simulink model "file_changed_port"  (R2021a)
settings: Solver=FixedStepDiscrete  StartTime=0.0  StopTime=10.0  RelTol=1e-3
CloseFcn:
  | try
  | rmdir slprj\ s
  | catch
  | end
  | try
  | folder_name = [bdroot '*'];
  | rmdir(folder_name,'s')
  | catch
  | end
  | try
  | file_temp_name = [bdroot '.slxc'];
  | delete(file_temp_name)
  | catch
  | end
  | clear folder_name file_temp_name
settings Model: Creator=Administrator  LastModifiedBy=Administrator
settings DataIOCC: SaveOutput=off  SignalLogging=off  DSMLogging=off  SaveTime=off  ReturnWorkspaceOutputs=off
settings OptimizationCC: DefaultParameterBehavior=Inlined  EnhancedBackFolding=on  PassReuseOutputArgsAs=Individual arguments  ZeroExternalMemoryAtStartup=off  ZeroInternalMemoryAtStartup=off  OptimizeBlockOrder=speed  DifferentSizesBufferReuse=on  OptimizationCustomize=off  EfficientTunableParamExpr=on
settings DebuggingCC: ParameterTunabilityLossMsg=error
settings SFSimCC: MATLABDynamicMemAlloc=off
settings RTWCC: SystemTargetFile=ert.tlc  GenCodeOnly=on  TemplateMakefile=ert_default_tmf  GenerateReport=on  LaunchReport=on
settings CodeAppCC: ForceParamTrailComments=on  IgnoreCustomStorageClasses=off  OperatorAnnotations=on  SimulinkDataObjDesc=on  SFDataObjDesc=on  InsertBlockDesc=on
settings ERTTargetCC: TargetLangStandard=C99 (ISO)  GenerateSampleERTMain=on  InlinedParameterPlacement=NonHierarchical  ERTCustomFileTemplate=example_file_process.tlc

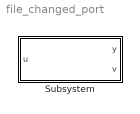
== system file_changed_port ==
  Subsystem : Subsystem  mask{gain=0, P=on}
      mask prompts: P "Sel"
      mask Callback P:
      | userdata = get(gcbh,'userdata');
      | state = get(gcbh,'P');
      | if ~strcmp(state,userdata)
      |         if strcmp(state,'on')
      |             replace_block([get(gcbh,'Parent') '/' get(gcbh, 'Name')],'Name', 'y','Outport','noprompt')
      |             set_param([gcb '/y'],'Port','1')
      |         end
      |         if strcmp(state,'off')
      |             replace_block([get(gcbh,'Parent') '/' get(gcbh, 'Name')],'Name', 'y','Terminator','noprompt')
      |         end
      | end
      | set(gcbh,'userdata',state);

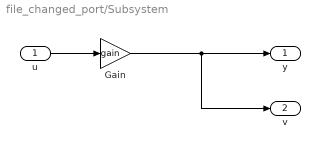
== system file_changed_port/Subsystem ==
  u : Inport
  Gain : Gain  Gain=gain
  y : Outport
  v : Outport  Port=2
  wires:
  u/1 -> Gain/1
  Gain/1 -> v/1, y/1
